simulink model "test"  (R2019b)
settings: Solver=VariableStepAuto  StartTime=0.0  StopTime=0.003  RelTol=1e-3
settings Model: Creator=andre  LastModifiedBy=Emanuel Pereira

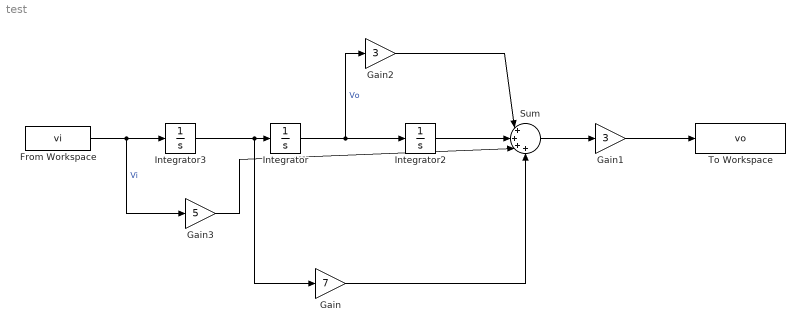
== system test ==
  From Workspace : FromWorkspace  VariableName=vi  SampleTime=0
  Gain : Gain  Gain=7
  Gain1 : Gain  Gain=3
  Gain2 : Gain  Gain=3
  Gain3 : Gain  Gain=5
  Integrator : Integrator
  Integrator2 : Integrator
  Integrator3 : Integrator
  Sum : Sum  Inputs=|++++
  To Workspace : ToWorkspace  VariableName=vo  SaveFormat=Timeseries  SampleTime=-1
  wires:
  From Workspace/1 -> Gain3/1, Integrator3/1  "Vi"
  Gain3/1 -> Sum/3
  Integrator3/1 -> Gain/1, Integrator/1
  Gain/1 -> Sum/4
  Integrator/1 -> Gain2/1, Integrator2/1  "Vo"
  Integrator2/1 -> Sum/2
  Gain2/1 -> Sum/1
  Sum/1 -> Gain1/1
  Gain1/1 -> To Workspace/1
